simulink model "Controller"  (R2017b)
settings: Solver=VariableStepAuto  StartTime=0.0  StopTime=10.0  RelTol=1e-3
libraries: nesl_utility x6
settings Model: Creator=Kalana  LastModifiedBy=Kalana

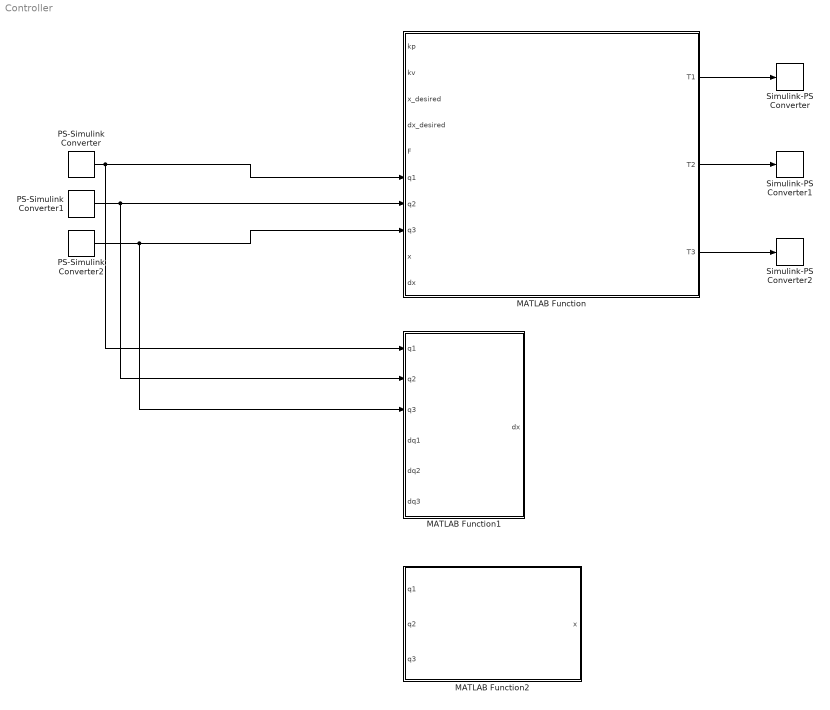
== system Controller ==
  MATLAB Function : MATLAB Function  TreatAsAtomicUnit=on
  MATLAB Function1 : MATLAB Function  TreatAsAtomicUnit=on
  MATLAB Function2 : MATLAB Function  TreatAsAtomicUnit=on
  PS-Simulink Converter : nesl_utility/PS-Simulink Converter  PhysicalDomain=network_engine_domain  SubClassName=ps_output  LeftPortType=input  RightPortType=output  PseudoPeriodic=off  Frequencies=[]  Unit=1  AffineConversion=off
  PS-Simulink Converter1 : nesl_utility/PS-Simulink Converter  PhysicalDomain=network_engine_domain  SubClassName=ps_output  LeftPortType=input  RightPortType=output  PseudoPeriodic=off  Frequencies=[]  Unit=1  AffineConversion=off
  PS-Simulink Converter2 : nesl_utility/PS-Simulink Converter  PhysicalDomain=network_engine_domain  SubClassName=ps_output  LeftPortType=input  RightPortType=output  PseudoPeriodic=off  Frequencies=[]  Unit=1  AffineConversion=off
  Simulink-PS Converter : nesl_utility/Simulink-PS Converter  PhysicalDomain=network_engine_domain  SubClassName=ps_input  LeftPortType=input  RightPortType=output  PseudoPeriodic=off  Frequencies=[]  NoiseDistribution=none  NoiseParameters=[]  Unit=1  AffineConversion=off  FilteringAndDerivatives=provide  SimscapeFilterOrder=1  InputFilterTimeConstant=0.001  UdotUserProvided=0
  Simulink-PS Converter1 : nesl_utility/Simulink-PS Converter  PhysicalDomain=network_engine_domain  SubClassName=ps_input  LeftPortType=input  RightPortType=output  PseudoPeriodic=off  Frequencies=[]  NoiseDistribution=none  NoiseParameters=[]  Unit=1  AffineConversion=off  FilteringAndDerivatives=provide  SimscapeFilterOrder=1  InputFilterTimeConstant=0.001  UdotUserProvided=0
  Simulink-PS Converter2 : nesl_utility/Simulink-PS Converter  PhysicalDomain=network_engine_domain  SubClassName=ps_input  LeftPortType=input  RightPortType=output  PseudoPeriodic=off  Frequencies=[]  NoiseDistribution=none  NoiseParameters=[]  Unit=1  AffineConversion=off  FilteringAndDerivatives=provide  SimscapeFilterOrder=1  InputFilterTimeConstant=0.001  UdotUserProvided=0
  wires:
  MATLAB Function/1(T1) -> Simulink-PS Converter/1
  MATLAB Function/2(T2) -> Simulink-PS Converter1/1
  MATLAB Function/3(T3) -> Simulink-PS Converter2/1
  PS-Simulink Converter/1 -> MATLAB Function1/1(q1), MATLAB Function/6(q1)
  PS-Simulink Converter1/1 -> MATLAB Function1/2(q2), MATLAB Function/7(q2)
  PS-Simulink Converter2/1 -> MATLAB Function1/3(q3), MATLAB Function/8(q3)

== matlab function Controller/MATLAB Function1 ==
  data: q1 input; dx output; q2 input; q3 input; dq1 input; dq2 input; dq3 input
function dx = Jacobian(q1, q2, q3, dq1, dq2, dq3)

dq = [ dq1;
       dq2;
       dq3];

JvEE =[-0.265*sind(q1)*cosd(q2-q3)-0.2*sind(q1)*cosd(q2)-0.1225*sind(q1)-0.0525*cosd(q1), -0.265*cosd(q1)*sind(q2-q3)-0.2*cosd(q1)*sind(q2),     0.265*cosd(q1)*sind(q2-q3) ;
       0,                                                                                 0.265*cosd(q2-q3)+0.2*cosd(q2),                        -0.265*cosd(q2-q3)         ;
       -0.265*cosd(q1)*cosd(q2-q3)-0.2*cosd(q1)*cosd(q2)-0.1225*cosd(q1)+0.0525*sind(q1), 0.265*sind(q1)*sind(q2-q3)+0.2*sind(q1)*sind(q2),      -0.265*sind(q1)*sind(q2-q3)]; 
   
dx = JvEE*dq;

== matlab function Controller/MATLAB Function ==
  data: kp input; kv input; x_desired input; dx_desired input; F input; T1 output; q1 input; q2 input; q3 input; x input; dx input; T2 output; T3 output
function [T1, T2, T3] = rightLegControl(kp, kv, x_desired, dx_desired, F, q1, q2, q3, x, dx)

g = [0    ;
     0    ;
     -9.8 ];

Mass_1 = [1.13919,  0,        0;
          0,        1.13919,  0;
          0,        0,        1.13919];

Iner_1 = [ 4703123.40e-09,     -3169987.54e-09,     210.39e-09;
           -3169987.54e-09,    4976200.05e-09,     -364.11e-09;
           210.39e-09,         -364.11e-09,         8601629.18e-09];

      
Mass_2 = [1.13671,  0,        0;
          0,        1.13671,  0;
          0,        0,        1.13671];

Iner_2 = [2565673.28e-09,      32.99e-09,           2839694.73e-09;
          32.99e-09,           12592746.15e-09,     -50.96e-09;
          2839694.73e-09,      -50.96e-09,          10643810.45e-09];

      
Mass_3 = [0.63820,  0,        0;
          0,        0.63820,  0;
          0,        0,        0.63280];
  
Iner_3 = [728680.81e-09,      -172.39e-09,        158.48e-09;
          -172.39e-09,        2618699.35e-09,     -3.33e-09;
          158.48e-09,         -3.33e-09,          2391085.66e-09];

      
Jv1 = [-0.05734*cos(q1)-0.05586*sin(q1),   0, 0;
       0,                                  0, 0;
       +0.05734*sin(q1)-0.05586*cos(q1)    0, 0];

Jw1 = [0, 0, 0;
       1, 0, 0;
       0, 0, 0];

   
Jv2 = [-0.100*sin(q1)*cos(q2)-0.0773*cos(q1)-0.1225*sin(q1),  -0.100*cos(q1)*sin(q2),     0;
       0,                                                     0.100*cos(q2),              0; 
       0.100*cos(q1)*cos(q2)+0.0773*sin(q1)-0.1225*cos(q1),   -0.100*sin(q1)*sin(q2),     0]; 
      
Jw2 = [0, 1, 0; 
       1, 0, 0; 
       0, 0, 0];
 
   
Jv3 = [-0.02559*sin(q1)*cos(q2-q3)-0.2*sin(q1)*cos(q2)-0.1225*sin(q1)-0.0525*cos(q1),  -0.02559*cos(q1)*sin(q2-q3)-0.2*cos(q1)*sin(q2),  0.02559*cos(q1)*sin(q2-q3) ;
       0,                                                                              0.02559*cos(q2-q3)+0.2*cos(q2),                   -0.02559*cos(q2-q3)         ;
       -0.02559*cos(q1)*cos(q2-q3)-0.2*cos(q1)*cos(q2)-0.1225*cos(q1)+0.0525*sin(q1),  0.02559*sin(q1)*sin(q2-q3)+0.2*sin(q1)*sin(q2),   -0.02559*sin(q1)*sin(q2-q3)];
      
Jw3 = [0, 1, -1;
       1, 0,  0;
       0, 0,  0];

   
JvEE =[-0.265*sin(q1)*cos(q2-q3)-0.2*sin(q1)*cos(q2)-0.1225*sin(q1)-0.0525*cos(q1), -0.265*cos(q1)*sin(q2-q3)-0.2*cos(q1)*sin(q2),     0.265*cos(q1)*sin(q2-q3) ;
       0,                                                                           0.265*cos(q2-q3)+0.2*cos(q2),                      -0.265*cos(q2-q3)         ;
       -0.265*cos(q1)*cos(q2-q3)-0.2*cos(q1)*cos(q2)-0.1225*cos(q1)+0.0525*sin(q1), 0.265*sin(q1)*sin(q2-q3)+0.2*sin(q1)*sin(q2),      -0.265*sin(q1)*sin(q2-q3)]; 
   

Mass_q = Jv1'*Mass_1*Jv1 + Jw1'*Iner_1*Jw1 + Jv2'*Mass_2*Jv2 + Jw2'*Iner_2*Jw2 + Jv3'*Mass_3*Jv3 + Jw3'*Iner_3*Jw3;

Mass_x = JvEE'*pinv(JvEE*inv(Mass_q)*JvEE');

Grav = Jv1'*M1*g + Jv2'*M2*g + Jv3'*M3*g;

Force = JvEE'*F;

torque = Mass_x(kp(x_desired - x) + kv(dx_desired - dx)) + Grav + Force;

T1 = torque(1);
T2 = torque(2);
T3 = torque(3);

== matlab function Controller/MATLAB Function2 ==
  data: q1 input; x output; q2 input; q3 input
function x = Kinematics(q1, q2, q3)

leg = [0.265;
       0;
       0;
       1];
   
Trans0_3 = [cosd(q1)*cosd(q2-q3),   cosd(q1)*sind(q2-q3),   -sind(q1),      0.2*cosd(q1)*cosd(q2)+0.1225*cosd(q1)-0.0525*sind(q1);
            sind(q2-q3),            -cosd(q2-q3),           0,              0.2*sind(q2);
            -sind(q1)*cosd(q2-q3),  -sind(q1)*sind(q2-q3),  -cosd(q1),      -0.2*sind(q1)*cosd(q2)-0.1225*sind(q1)-0.0525*cosd(q1);
            0,                      0,                      0,              1];
        
x_temp = Trans0_3*leg;

x = x_temp(1:3);
